simulink model "saturn_ib_stack_test"  (Simulink 6.2)
settings: Solver=ode4  SolverMode=SingleTasking  StartTime=-20.0  StopTime=620  FixedStep=0.005  RelTol=1e-3
values from neighbouring files (symbols this model uses):
  A_z_deg = 82.8200    (= 82.82)    [AS205_presettings.m]
  BN_1_sec = 14.4    [AS205_presettings.m]
  DeltaV_b_mps = 7.2381    [AS205_presettings.m]
  epsilon_2_sec = 15.0    (= 15)    [AS205_presettings.m]
  epsilon_prime_sec = 3.0    (= 3)    [AS205_presettings.m]
  i_deg = 28.89597    [AS205_presettings.m]
  lambda_0_deg = 102.32900    (= 102.329)    [AS205_presettings.m]
  lambda_L_deg = -80.561141    [AS205_presettings.m]
  pad_roll_L_deg = 100.0    (= 100)    [AS205_presettings.m]
  phi_L_deg = 28.521963    [AS205_presettings.m]
  phi_L_prime_deg = 28.360795    [AS205_presettings.m]
  R_L_m = 6373385.0    (= 6373385)    [AS205_presettings.m]
  R_T_m = 6570774.0    (= 6570774)    [AS205_presettings.m]
  T3_FM_sec = 6.08    [AS205_presettings.m]
  T_HSL_sec = 5.0    (= 5)    [AS205_presettings.m]
  Theta_T_deg = 0.000    (= 0)    [AS205_presettings.m]
  V_T_mps = 7780.976    [AS205_presettings.m]
  Xdotdot_VGT_mps2 = -9.251    [AS205_presettings.m]
undefined symbols (not defined in the file or in its folder): e0_0, e1_0, e2_0, e3_0, m, s
libraries: simulink x99, aerolibconvert x83, aerolibutil x63, aerolibtransform2 x34, aerolibasang x2, aerolibatmos2 x2, aerolib6dofsys x2
(part 7 of 7)

== system saturn_ib_stack_test/Saturn_IB_Stack/Saturn Instrument Unit (IU)/LVDA / LVDC/LVDC Iterative Guidance Mode/Position Correction Terms ==
  note: Enable Chi-tilde steering mode when T_3_i countdown
      | is near cutoff.  This is described in EDD section
      | 4.4.2.4, "Terminal Steering and Cutoff".
  J_prime_3 : Inport  Port=1  LatchInput=off
  tau_3_sec : Inport  Port=2  LatchInput=off
  T_3_i_sec : Inport  Port=3  LatchInput=off
  L_1 : Inport  Port=4  LatchInput=off
  J_1 : Inport  Port=5  LatchInput=off
  T_1_i_sec : Inport  Port=6  LatchInput=off
  S_1 : Inport  Port=7  LatchInput=off
  P_1 : Inport  Port=8  LatchInput=off
  Q_1 : Inport  Port=9  LatchInput=off
  U_1 : Inport  Port=10  LatchInput=off
  R_V_bar_m : Inport  Port=11  LatchInput=off
  V_V_bar_mps : Inport  Port=12  LatchInput=off
  G_star_V_bar_mps2 : Inport  Port=13  LatchInput=off
  T_star : Inport  Port=14  LatchInput=off
  L_3 : Inport  Port=15  LatchInput=off
  DeltaL_3 : Inport  Port=16  LatchInput=off
  Chi_z_tilde : Inport  Port=17  LatchInput=off
  Chi_y_tilde : Inport  Port=18  LatchInput=off
  Compare To Constant : simulink/Logic and Bit Operations/Compare To Constant  relop=<=  const=epsilon_2_sec  LogicOutDataTypeMode=boolean  ZeroCross=off
  Ground : Ground
  "Position Correction Terms - part 1 K_3, K_4 (Eqns. 4.4.51-67)" : Subsystem
  "Position Correction Terms - part 2 K_1, K_2 (Eqns. 4.4.68-80)" : Subsystem
  Switch{,1..3} (4 alike) : Switch  Criteria=u2 ~= 0
  K_1 : Outport
  K_2 : Outport  Port=2
  K_3 : Outport  Port=3
  K_4 : Outport  Port=4
  L_y : Outport  Port=5
  C_2 : Outport  Port=6
  C_4 : Outport  Port=7
  wires:
  DeltaL_3/1 -> "Position Correction Terms - part 1 K_3, K_4 (Eqns. 4.4.51-67)"/2(Delta_L_3)
  J_prime_3/1 -> "Position Correction Terms - part 1 K_3, K_4 (Eqns. 4.4.51-67)"/1(J_prime_3)
  tau_3_sec/1 -> "Position Correction Terms - part 2 K_1, K_2 (Eqns. 4.4.68-80)"/12(tau_3_sec), "Position Correction Terms - part 1 K_3, K_4 (Eqns. 4.4.51-67)"/3(tau_3_sec)
  L_1/1 -> "Position Correction Terms - part 1 K_3, K_4 (Eqns. 4.4.51-67)"/5(L_1)
  J_1/1 -> "Position Correction Terms - part 1 K_3, K_4 (Eqns. 4.4.51-67)"/6(J_1)
  S_1/1 -> "Position Correction Terms - part 1 K_3, K_4 (Eqns. 4.4.51-67)"/8(S_1)
  L_3/1 -> "Position Correction Terms - part 1 K_3, K_4 (Eqns. 4.4.51-67)"/9(L_3), "Position Correction Terms - part 2 K_1, K_2 (Eqns. 4.4.68-80)"/11(L_3)
  Q_1/1 -> "Position Correction Terms - part 1 K_3, K_4 (Eqns. 4.4.51-67)"/10(Q_1)
  R_V_bar_m/1 -> "Position Correction Terms - part 2 K_1, K_2 (Eqns. 4.4.68-80)"/16(R_V_bar_m), "Position Correction Terms - part 1 K_3, K_4 (Eqns. 4.4.51-67)"/11(R_V_bar_m)
  V_V_bar_mps/1 -> "Position Correction Terms - part 1 K_3, K_4 (Eqns. 4.4.51-67)"/12(V_V_bar_mps), "Position Correction Terms - part 2 K_1, K_2 (Eqns. 4.4.68-80)"/17(V_V_bar_mps)
  T_star/1 -> "Position Correction Terms - part 2 K_1, K_2 (Eqns. 4.4.68-80)"/19(T_star), "Position Correction Terms - part 1 K_3, K_4 (Eqns. 4.4.51-67)"/14(T_star)
  G_star_V_bar_mps2/1 -> "Position Correction Terms - part 2 K_1, K_2 (Eqns. 4.4.68-80)"/18(G_star_V_bar_mps2), "Position Correction Terms - part 1 K_3, K_4 (Eqns. 4.4.51-67)"/13(G_star_V_bar_mps2)
  T_3_i_sec/1 -> "Position Correction Terms - part 1 K_3, K_4 (Eqns. 4.4.51-67)"/4(T_3_i_sec), "Position Correction Terms - part 2 K_1, K_2 (Eqns. 4.4.68-80)"/13(T_3_i_sec), [T_3_i]
  T_1_i_sec/1 -> "Position Correction Terms - part 1 K_3, K_4 (Eqns. 4.4.51-67)"/7(T_1_i_sec), "Position Correction Terms - part 2 K_1, K_2 (Eqns. 4.4.68-80)"/14(T_1_i_sec)
  Chi_z_tilde/1 -> "Position Correction Terms - part 2 K_1, K_2 (Eqns. 4.4.68-80)"/20(Chi_z_tilde), "Position Correction Terms - part 1 K_3, K_4 (Eqns. 4.4.51-67)"/15(Chi_z)
  "Position Correction Terms - part 2 K_1, K_2 (Eqns. 4.4.68-80)"/1(K_1) -> Switch2/3
  "Position Correction Terms - part 1 K_3, K_4 (Eqns. 4.4.51-67)"/7(Q_y) -> "Position Correction Terms - part 2 K_1, K_2 (Eqns. 4.4.68-80)"/7(Q_y)
  "Position Correction Terms - part 2 K_1, K_2 (Eqns. 4.4.68-80)"/2(K_2) -> Switch3/3
  "Position Correction Terms - part 1 K_3, K_4 (Eqns. 4.4.51-67)"/8(K_3) -> "Position Correction Terms - part 2 K_1, K_2 (Eqns. 4.4.68-80)"/9(K_3), Switch/3
  "Position Correction Terms - part 1 K_3, K_4 (Eqns. 4.4.51-67)"/9(K_4) -> "Position Correction Terms - part 2 K_1, K_2 (Eqns. 4.4.68-80)"/10(K_4), Switch1/3
  "Position Correction Terms - part 1 K_3, K_4 (Eqns. 4.4.51-67)"/1(J_3) -> "Position Correction Terms - part 2 K_1, K_2 (Eqns. 4.4.68-80)"/1(J_3)  "J_3"
  "Position Correction Terms - part 1 K_3, K_4 (Eqns. 4.4.51-67)"/2(S_3) -> "Position Correction Terms - part 2 K_1, K_2 (Eqns. 4.4.68-80)"/2(S_3)  "S_3"
  "Position Correction Terms - part 1 K_3, K_4 (Eqns. 4.4.51-67)"/3(Q_3) -> "Position Correction Terms - part 2 K_1, K_2 (Eqns. 4.4.68-80)"/3(Q_3)
  "Position Correction Terms - part 1 K_3, K_4 (Eqns. 4.4.51-67)"/4(L_y) -> "Position Correction Terms - part 2 K_1, K_2 (Eqns. 4.4.68-80)"/4(L_y), L_y/1  "L_y"
  "Position Correction Terms - part 1 K_3, K_4 (Eqns. 4.4.51-67)"/5(J_y) -> "Position Correction Terms - part 2 K_1, K_2 (Eqns. 4.4.68-80)"/5(J_y)
  "Position Correction Terms - part 1 K_3, K_4 (Eqns. 4.4.51-67)"/6(S_y) -> "Position Correction Terms - part 2 K_1, K_2 (Eqns. 4.4.68-80)"/6(S_y)
  P_1/1 -> "Position Correction Terms - part 2 K_1, K_2 (Eqns. 4.4.68-80)"/15(P_1)
  Chi_y_tilde/1 -> "Position Correction Terms - part 2 K_1, K_2 (Eqns. 4.4.68-80)"/8(Chi_y_tilde)
  U_1/1 -> "Position Correction Terms - part 2 K_1, K_2 (Eqns. 4.4.68-80)"/21(U_1)
  "Position Correction Terms - part 2 K_1, K_2 (Eqns. 4.4.68-80)"/3(C_2) -> C_2/1
  "Position Correction Terms - part 2 K_1, K_2 (Eqns. 4.4.68-80)"/4(C_4) -> C_4/1
  Ground/1 -> Switch/1, Switch1/1, Switch2/1, Switch3/1
  Switch/1 -> K_3/1
  Switch1/1 -> K_4/1
  [T_3_i] -> Compare To Constant/1
  Compare To Constant/1 -> Switch/2, Switch1/2, Switch2/2, Switch3/2
  Switch2/1 -> K_1/1
  Switch3/1 -> K_2/1

== system saturn_ib_stack_test/Saturn_IB_Stack/Saturn Instrument Unit (IU)/LVDA / LVDC/LVDC Iterative Guidance Mode/SMCY ==
  Chi_y : Inport  Port=1  LatchInput=off
  Xdotdot_m : Inport  Port=2  LatchInput=off
  Zdotdot_m : Inport  Port=3  LatchInput=off
  Enable : EnablePort
  Add17 : Sum  Inputs=+-  OutScaling=2^-10
  Add19 : Sum  OutScaling=2^-10
  Add20 : Sum  Inputs=+-  OutScaling=2^-10
  Chi_y_last : Memory  InheritSampleTime=on
  Chi_y_last2 : Memory  InheritSampleTime=on
  Constant9 : Constant  Value=delta_T_sec/pi
  Divide6 : Product  Inputs=**/  OutScaling=2^-10
  Gain1 : Gain  Gain=0.5
  Product18 : Product  RndMeth=Zero
  Product19 : Product  RndMeth=Zero
  SMCG (Y-Axis) : Gain  Gain=0.03
  SMCY : Memory  Orientation=left  InheritSampleTime=on
  Sum2 : Sum  Inputs=|++  SampleTime=1.6
  Sum5 : Sum  Inputs=++|
  Trigonometric Function6 : Trigonometry  Operator=tan
  pirads to radians : Gain  Gain=pi
  SMCY_rad : Outport
  wires:
  SMCY/1 -> Sum2/2, Add20/2
  Sum2/1 -> SMCY/1, pirads to radians/1
  Chi_y_last/1 -> Sum5/2, Chi_y_last2/1
  Chi_y_last2/1 -> Sum5/1
  SMCG (Y-Axis)/1 -> Sum2/1
  Add20/1 -> Trigonometric Function6/1
  Divide6/1 -> SMCG (Y-Axis)/1
  Trigonometric Function6/1 -> Product19/1, Product18/1
  Xdotdot_m/1 -> Add17/1, Product18/2
  Zdotdot_m/1 -> Add19/1, Product19/2
  Product18/1 -> Add19/2
  Product19/1 -> Add17/2
  Constant9/1 -> Divide6/1
  Add19/1 -> Divide6/2
  Add17/1 -> Divide6/3
  Sum5/1 -> Gain1/1
  Gain1/1 -> Add20/1
  Chi_y/1 -> Chi_y_last/1
  pirads to radians/1 -> SMCY_rad/1

== system saturn_ib_stack_test/Saturn_IB_Stack/Saturn Instrument Unit (IU)/LVDA / LVDC/LVDC Iterative Guidance Mode/SMCZ ==
  Chi_z : Inport  Port=1  LatchInput=off
  Ydotdot_m : Inport  Port=2  LatchInput=off
  FoverM : Inport  Port=3  LatchInput=off
  Enable : EnablePort
  Add16 : Sum  Inputs=+-  OutScaling=2^-10
  Add18 : Sum  Inputs=+-  OutScaling=2^-10
  Chi_z_last : Memory  InheritSampleTime=on
  Chi_z_last2 : Memory  InheritSampleTime=on
  Constant8 : Constant  Value=delta_T_sec/pi
  Divide5 : Product  Inputs=**/  OutScaling=2^-10
  Divide7 : Product  Inputs=**  OutScaling=2^-10
  Gain : Gain  Gain=0.5
  Math Function8 : Math  Operator=reciprocal  SaturateOnIntegerOverflow=on
  SMCG : Gain  Gain=0.03
  SMCZ : Memory  Orientation=left  InheritSampleTime=on
  SinCos2 : aerolibutil/SinCos
  Sum3 : Sum  Inputs=|++  SampleTime=1.6
  Sum4 : Sum  Inputs=++|
  pirads to radians : Gain  Gain=pi
  SMCZ_rad : Outport
  wires:
  SMCZ/1 -> Sum3/2, Add16/2
  Sum3/1 -> SMCZ/1, pirads to radians/1
  Chi_z_last2/1 -> Sum4/1
  Sum4/1 -> Gain/1
  SMCG/1 -> Sum3/1
  Gain/1 -> Add16/1
  Add16/1 -> SinCos2/1
  Chi_z_last/1 -> Chi_z_last2/1, Sum4/2
  Divide5/1 -> SMCG/1
  Constant8/1 -> Divide5/1
  SinCos2/2 -> Divide5/3
  Add18/1 -> Divide5/2
  SinCos2/1 -> Add18/1
  Divide7/1 -> Add18/2
  Math Function8/1 -> Divide7/2
  Chi_z/1 -> Chi_z_last/1
  Ydotdot_m/1 -> Divide7/1
  FoverM/1 -> Math Function8/1
  pirads to radians/1 -> SMCZ_rad/1

== system saturn_ib_stack_test/Saturn_IB_Stack/Saturn Instrument Unit (IU)/LVDA / LVDC/LVDC Iterative Guidance Mode/Vector Display2 ==
  In1 : Inport  Port=1  LatchInput=off
  Demux5 : Demux  Outputs=3
  R_V_X : Display
  R_V_Y : Display
  R_V_Z : Display
  wires:
  Demux5/1 -> R_V_X/1
  Demux5/2 -> R_V_Y/1
  Demux5/3 -> R_V_Z/1
  In1/1 -> Demux5/1

== system saturn_ib_stack_test/Saturn_IB_Stack/Saturn Instrument Unit (IU)/LVDA / LVDC/LVDC S-Frame Position & Velocity Calculations/Estimated Gravitational Acceleration (Eqns. 4.3.6-12) ==
  note: Eqn. 4.3.6
  note: Eqn. 4.3.7
  note: Eqn. 4.3.12
  note: Eqn. 4.3.10
  note: Eqn. 4.3.11
  note: Mux outputs:
      | u(1)  X_S
      | u(2)  Y_S
      | u(3)  Z_S
      | u(4)  Y_G_bar
      | u(5)  R_m
      | u(6)  a_e/R_m
      | u(7)  Y_G/R_m
  XYZ_S_m : Inport  Port=1  LatchInput=off
  A_z_deg : Inport  Port=2  LatchInput=off
  phi_L_deg : Inport  Port=3  LatchInput=off
  2J : Gain  Gain=2.0*J
  Add : Sum  OutScaling=2^-10
  Add1 : Sum  OutScaling=2^-10
  Add2 : Sum  OutScaling=2^-10
  Angle Conversion : aerolibconvert/Angle Conversion  IU=deg  OU=rad
  Angle Conversion1 : aerolibconvert/Angle Conversion  IU=deg  OU=rad
  Constant : Constant  Value=-mu  OutDataTypeMode=double
  Constant1 : Constant  Value=-mu  OutDataTypeMode=double
  Divide : Product  Inputs=*/  OutScaling=2^-10
  Divide1 : Product  Inputs=*/  OutScaling=2^-10
  Divide2 : Product  Inputs=***/  OutScaling=2^-10
  Math Function : Math  Operator=square  SaturateOnIntegerOverflow=on
  Mux : Mux  Inputs=5
  Mux1 : Mux  Inputs=5
  Mux2 : Mux  Inputs=3
  P_34 : Fcn  Expr=H*u(6)*(15.0*u(7)^2-3.0) + (D/7.0)*u(6)^2*u(7)*(12.0-28.0*u(7)^2)
  Product : Product  RndMeth=Zero
  Product1 : Product  RndMeth=Zero
  Product2 : Product  RndMeth=Zero
  R^2 : Fcn  Expr=u(1)^2
  R^3 : Fcn  Expr=u(1)^3
  R_m : Fcn  Expr=sqrt(u(1)^2+u(2)^2+u(3)^2)
  S_34 : Fcn  Expr=H*u(6)^3*u(7)*(3-7*u(7)^2)+(D/7.0)*u(6)^4*(3.0-42*u(7)^2+63*u(7)^4)
  S_term : Fcn  Expr=1.0 + J*u(6)^2*(1.0-5.0*u(7)^2)
  SinCos1 : aerolibutil/SinCos
  SinCos2 : aerolibutil/SinCos
  X : Fcn  Expr=-u(6)
  Y : Fcn  Expr=u(7)*u(4)
  Y1 : Fcn  Expr=-u(7)*u(5)
  Y_G : Fcn  Expr=-u(1)*u(6)+u(2)*u(7)*u(4)-u(3)*u(7)*u(5)
  aaa : Fcn  Expr=a_e_m/u(1)
  Y_G_m : Outport
  G_S_bar_mps2 : Outport  Port=2  PortDimensions=3
  wires:
  A_z_deg/1 -> Angle Conversion/1
  Angle Conversion/1 -> SinCos1/1
  phi_L_deg/1 -> Angle Conversion1/1
  Angle Conversion1/1 -> SinCos2/1
  XYZ_S_m/1 -> Mux/1, Mux1/1, Product2/1
  SinCos1/1 -> Mux/2
  SinCos1/2 -> Mux/3
  SinCos2/1 -> Mux/4
  SinCos2/2 -> Mux/5
  Mux/1 -> Y_G/1, R_m/1, X/1, Y/1, Y1/1
  Y_G/1 -> Y_G_m/1, Mux1/2, Divide/1
  R_m/1 -> Mux1/3, Divide/2, R^3/1, R^2/1, aaa/1
  Mux1/1 -> P_34/1, S_term/1, S_34/1
  aaa/1 -> Mux1/4, Math Function/1
  Divide/1 -> Mux1/5, 2J/1
  Constant/1 -> Divide1/1
  R^3/1 -> Divide1/2
  S_term/1 -> Add/2
  Add/1 -> Product/1
  Divide1/1 -> Product/2
  Constant1/1 -> Divide2/1
  Math Function/1 -> Divide2/2
  X/1 -> Mux2/1
  Y/1 -> Mux2/2
  Y1/1 -> Mux2/3
  Mux2/1 -> Product1/2
  Divide2/1 -> Product1/1  "P"
  Product/1 -> Product2/2  "S"
  Product2/1 -> Add1/1
  Product1/1 -> Add1/2
  Add1/1 -> G_S_bar_mps2/1
  R^2/1 -> Divide2/4
  Add2/1 -> Divide2/3
  2J/1 -> Add2/1
  P_34/1 -> Add2/2
  S_34/1 -> Add/1

== system saturn_ib_stack_test/Saturn_IB_Stack/Saturn Instrument Unit (IU)/LVDA / LVDC/LVDC S-Frame Position & Velocity Calculations/Initial Position and Velocity (Eqns. 3.4.3-4) ==
  R_L_m : Inport  Port=1  PortDimensions=1  LatchInput=off
  A_z_deg : Inport  Port=2  LatchInput=off
  phi_L_deg : Inport  Port=3  LatchInput=off
  phi_L_prime_deg : Inport  Port=4  LatchInput=off
  Add : Sum  Inputs=+-  OutScaling=2^-10
  Angle Conversion : aerolibconvert/Angle Conversion  IU=deg  OU=rad
  Angle Conversion1 : aerolibconvert/Angle Conversion  IU=deg  OU=rad
  Angle Conversion2 : aerolibconvert/Angle Conversion  IU=deg  OU=rad
  Fcn : Fcn  Expr=u(1)*u(7)
  Fcn1 : Fcn  Expr=u(1)*u(6)*u(2)
  Fcn2 : Fcn  Expr=-u(1)*u(6)*u(3)
  Fcn3 : Fcn  Expr=0.0
  Fcn4 : Fcn  Expr=u(1)*omega_E_rps*pi*u(9)*u(3)
  Fcn5 : Fcn  Expr=u(1)*omega_E_rps*pi*u(9)*u(2)
  Mux : Mux  Inputs=9
  Mux1 : Mux  Inputs=3
  Mux2 : Mux  Inputs=3
  SinCos{1..4} (4 alike) : aerolibutil/SinCos
  R_S_0_m : Outport
  V_S_0_mps : Outport  Port=2
  wires:
  A_z_deg/1 -> Angle Conversion/1
  Angle Conversion/1 -> SinCos1/1
  phi_L_deg/1 -> Angle Conversion1/1
  Angle Conversion1/1 -> SinCos2/1, Add/1
  R_L_m/1 -> Mux/1
  SinCos1/1 -> Mux/2
  SinCos1/2 -> Mux/3
  SinCos2/1 -> Mux/4
  SinCos2/2 -> Mux/5
  phi_L_prime_deg/1 -> Angle Conversion2/1
  Angle Conversion2/1 -> Add/2, SinCos4/1
  Add/1 -> SinCos3/1
  SinCos3/1 -> Mux/6
  SinCos3/2 -> Mux/7
  Fcn/1 -> Mux1/1
  Fcn1/1 -> Mux1/2
  Fcn2/1 -> Mux1/3
  Mux/1 -> Fcn/1, Fcn1/1, Fcn2/1, Fcn3/1, Fcn4/1, Fcn5/1
  Mux1/1 -> R_S_0_m/1
  Fcn3/1 -> Mux2/1
  Fcn4/1 -> Mux2/2
  Fcn5/1 -> Mux2/3
  Mux2/1 -> V_S_0_mps/1
  SinCos4/1 -> Mux/8
  SinCos4/2 -> Mux/9

== system saturn_ib_stack_test/Saturn_IB_Stack/Saturn Instrument Unit (IU)/LVDA / LVDC/LVDC S-Frame Position & Velocity Calculations/Position and Velocity Calculation (S-Frame) (Eqns. 4.3.1-5) ==
  note: Eqn. 4.2.10
  note: Eqn 4.2.9
  note: This needs to be revised to
      | compute outputs more closely
      | based on the EDD.
  XYZdot_m_mps : Inport  Port=1  SampleTime=1.6  LatchInput=off
  XYZdotdot_Sg_mps2 : Inport  Port=2  LatchInput=off
  XYZ_0_m : Inport  Port=3  LatchInput=off
  XYZdot_0_mps : Inport  Port=4  LatchInput=off
  Delta_T_sec : Inport  Port=5  LatchInput=off
  TGRR_bias_sec : Inport  Port=6  LatchInput=off
  Gain3 : Gain  Gain=1 / delta_T_sec
  Math Function3 : Math  Operator=sqrt  SaturateOnIntegerOverflow=on
  Math Function4 : Math  Operator=square  SaturateOnIntegerOverflow=on
  Memory2 : Memory  X0=[-0.5 0.0 0.0]  InheritSampleTime=on
  Product18 : Product  Multiplication=Matrix(*)  RndMeth=Zero
  Product6 : Product  Multiplication=Matrix(*)  RndMeth=Zero
  Sum : Sum  Inputs=|+-
  Sum of Elements1 : Sum  Inputs=+  OutScaling=2^-10
  Switch{1..3,5} (4 alike) : Switch  Criteria=u2 ~= 0
  T_1_i_sec : DataStoreMemory  DataStoreName=XYZdot_Sg_mps  InitialValue=[0.0 0.0 0.0]  DataType=double
  Terminator{,1..4} (5 alike) : Terminator
  tau_1_sec : DataStoreMemory  DataStoreName=XYZ_S_m  InitialValue=[0.0 0.0 0.0]  DataType=double
  XYZ_S_m : Outport  SampleTime=1.6
  XYZdot_S_mps : Outport  Port=2  PortDimensions=3  SampleTime=1.6
  A_m_bar_mps2 : Outport  Port=3  PortDimensions=3  SampleTime=1.6
  FoverM_mps2 : Outport  Port=4  PortDimensions=1  SampleTime=1.6
  wires:
  XYZdotdot_Sg_mps2/1 -> Terminator4/1
  XYZdot_m_mps/1 -> Memory2/1, Sum/1
  Sum of Elements1/1 -> Math Function3/1
  Math Function4/1 -> Sum of Elements1/1
  Math Function3/1 -> FoverM_mps2/1
  Memory2/1 -> Sum/2
  Sum/1 -> Gain3/1
  Gain3/1 -> Math Function4/1, A_m_bar_mps2/1
  [S_IVB_Xe_m] -> Switch5/1
  [bStageSep] -> Switch5/2
  Switch5/1 -> Product18/2
  [MES_DCM] -> Product18/1
  Product18/1 -> XYZ_S_m/1
  [S_IVB_Ve_mps] -> Switch1/1
  [bStageSep] -> Switch1/2
  Switch1/1 -> Product6/2
  [MES_DCM] -> Product6/1
  Product6/1 -> XYZdot_S_mps/1
  XYZ_0_m/1 -> Terminator/1
  TGRR_bias_sec/1 -> Terminator1/1
  XYZdot_0_mps/1 -> Terminator2/1
  Delta_T_sec/1 -> Terminator3/1
  Switch3/1 -> Switch5/3
  [bLiftoff] -> Switch3/2
  [bLiftoff] -> Switch2/2
  Switch2/1 -> Switch1/3
  [Xe_m] -> Switch3/1
  [PAD_Xe_m] -> Switch3/3
  [PAD_Ve_mps] -> Switch2/3
  [Ve_mps] -> Switch2/1

== system saturn_ib_stack_test/Saturn_IB_Stack/Saturn Instrument Unit (IU)/LVDA / LVDC/LVDC S-Frame Position & Velocity Calculations/Reciprocal Acceleration Filter (EDD eqn. 4.2.11) ==
  A_S_mps2 : Inport  Port=1  DataType=double  LatchInput=off
  Enable : EnablePort
  +/- 0.25 sec^2/m : Saturate  UpperLimit=inf  LowerLimit=4.00
  MF2 : Memory  X0=0.135  InheritSampleTime=on
  MF3 : Memory  X0=0.135  InheritSampleTime=on
  MF4 : Memory  X0=0.135  InheritSampleTime=on
  MFK : Constant  Value=[0.0120948 0.0213339 -0.0261577 -0.00526684 2.80483 -2.85880 1.24933 -0.197360]
  MFS{1..4} (4 alike) : Memory  X0=0.135  InheritSampleTime=on
  Math Function5 : Math  Operator=reciprocal  SaturateOnIntegerOverflow=on
  Mux1 : Mux  Inputs=8
  Product1 : Product  RndMeth=Zero
  Sum of Elements : Sum  Inputs=+  OutScaling=2^-10
  MF_S : Outport
  wires:
  MFS2/1 -> MFS3/1, Mux1/6
  MFS1/1 -> MFS2/1, Mux1/5
  MFS3/1 -> MFS4/1, Mux1/7
  MF2/1 -> MF3/1, Mux1/2
  MF3/1 -> MF4/1, Mux1/3
  Mux1/1 -> Product1/1
  MFK/1 -> Product1/2
  Product1/1 -> Sum of Elements/1
  MF4/1 -> Mux1/4
  MFS4/1 -> Mux1/8
  Sum of Elements/1 -> MFS1/1, MF_S/1
  A_S_mps2/1 -> +/- 0.25 sec^2/m/1
  Math Function5/1 -> MF2/1, Mux1/1
  +/- 0.25 sec^2/m/1 -> Math Function5/1

== system saturn_ib_stack_test/Saturn_IB_Stack/Saturn Instrument Unit (IU)/LVDA / LVDC/T1 Timer/Timer Initialization ==
  In1 : Inport  Port=1  LatchInput=off
  Trigger : TriggerPort
  Data Store Write : DataStoreWrite  DataStoreName=A  SampleTime=-1
  wires:
  In1/1 -> Data Store Write/1

== system saturn_ib_stack_test/Saturn_IB_Stack/Saturn Instrument Unit (IU)/LVDA / LVDC/T2 Timer/Timer Initialization ==
  In1 : Inport  Port=1  LatchInput=off
  Trigger : TriggerPort
  Data Store Write : DataStoreWrite  DataStoreName=A  SampleTime=-1
  wires:
  In1/1 -> Data Store Write/1

== system saturn_ib_stack_test/Saturn_IB_Stack/Saturn Instrument Unit (IU)/LVDA / LVDC/T3 Timer/Timer Initialization ==
  In1 : Inport  Port=1  LatchInput=off
  Trigger : TriggerPort
  Data Store Write : DataStoreWrite  DataStoreName=A  SampleTime=-1
  wires:
  In1/1 -> Data Store Write/1

== system saturn_ib_stack_test/Saturn_IB_Stack/Saturn Instrument Unit (IU)/LVDA / LVDC/T4 Timer/Timer Initialization ==
  In1 : Inport  Port=1  LatchInput=off
  Trigger : TriggerPort
  Data Store Write : DataStoreWrite  DataStoreName=A  SampleTime=-1
  wires:
  In1/1 -> Data Store Write/1

== system saturn_ib_stack_test/Saturn_IB_Stack/On Pad/Initial Conditions/MES Transform/MES Transform/E-Frame to s-Frame (MES matrix) ==
  note: u(1)  sin Az
      | u(2)  sin Phi_L
      | u(3)  sin Theta_E
      | u(4)  cos Az
      | u(5)  cos Phi_L
      | u(6)  cos Theta_E
  note: Eqn 2.3.10
  Az phi_L Theta_E : Inport  Port=1  LatchInput=off
  11 : Fcn  Expr=u(5)*u(6)
  12 : Fcn  Expr=u(5)*u(3)
  13 : Fcn  Expr=u(2)
  21 : Fcn  Expr=u(2)*u(1)*u(6)-u(4)*u(3)
  22 : Fcn  Expr=u(2)*u(1)*u(3)+u(4)*u(6)
  23 : Fcn  Expr=-u(5)*u(1)
  31 : Fcn  Expr=-u(2)*u(4)*u(6)-u(1)*u(3)
  32 : Fcn  Expr=-u(2)*u(4)*u(3)+u(1)*u(6)
  33 : Fcn  Expr=u(5)*u(4)
  Mux : Mux  Inputs=2
  Mux2 : Mux  Inputs=9
  Reshape 9x1->3x3 : simulink/Math Operations/Reshape  OutputDimensionality=Customize  OutputDimensions=[3,3]
  SinCos3 : aerolibutil/SinCos
  DCM : Outport  InitialOutput=0
  wires:
  33/1 -> Mux2/9
  22/1 -> Mux2/5
  11/1 -> Mux2/1
  Mux2/1 -> Reshape 9x1->3x3/1
  Reshape 9x1->3x3/1 -> DCM/1
  Mux/1 -> 22/1, 11/1, 21/1, 31/1, 12/1, 32/1, 13/1, 33/1, 23/1
  23/1 -> Mux2/8
  13/1 -> Mux2/7
  32/1 -> Mux2/6
  12/1 -> Mux2/4
  31/1 -> Mux2/3
  21/1 -> Mux2/2
  Az phi_L Theta_E/1 -> SinCos3/1
  SinCos3/1 -> Mux/1
  SinCos3/2 -> Mux/2

== system saturn_ib_stack_test/Saturn_IB_Stack/S-IB Stage/H-1 Engine Cluster/Engine 1/Triggered Timer/Timer Initialization ==
  In1 : Inport  Port=1  LatchInput=off
  Trigger : TriggerPort
  Data Store Write : DataStoreWrite  DataStoreName=A  SampleTime=-1
  wires:
  In1/1 -> Data Store Write/1

== system saturn_ib_stack_test/Saturn_IB_Stack/S-IB Stage/H-1 Engine Cluster/Engine 2/Triggered Timer/Timer Initialization ==
  In1 : Inport  Port=1  LatchInput=off
  Trigger : TriggerPort
  Data Store Write : DataStoreWrite  DataStoreName=A  SampleTime=-1
  wires:
  In1/1 -> Data Store Write/1

== system saturn_ib_stack_test/Saturn_IB_Stack/S-IB Stage/H-1 Engine Cluster/Engine 3/Triggered Timer/Timer Initialization ==
  In1 : Inport  Port=1  LatchInput=off
  Trigger : TriggerPort
  Data Store Write : DataStoreWrite  DataStoreName=A  SampleTime=-1
  wires:
  In1/1 -> Data Store Write/1

== system saturn_ib_stack_test/Saturn_IB_Stack/S-IB Stage/H-1 Engine Cluster/Engine 4/Triggered Timer/Timer Initialization ==
  In1 : Inport  Port=1  LatchInput=off
  Trigger : TriggerPort
  Data Store Write : DataStoreWrite  DataStoreName=A  SampleTime=-1
  wires:
  In1/1 -> Data Store Write/1

== system saturn_ib_stack_test/Saturn_IB_Stack/S-IB Stage/H-1 Engine Cluster/Engine 5/Triggered Timer/Timer Initialization ==
  In1 : Inport  Port=1  LatchInput=off
  Trigger : TriggerPort
  Data Store Write : DataStoreWrite  DataStoreName=A  SampleTime=-1
  wires:
  In1/1 -> Data Store Write/1

== system saturn_ib_stack_test/Saturn_IB_Stack/S-IB Stage/H-1 Engine Cluster/Engine 6/Triggered Timer/Timer Initialization ==
  In1 : Inport  Port=1  LatchInput=off
  Trigger : TriggerPort
  Data Store Write : DataStoreWrite  DataStoreName=A  SampleTime=-1
  wires:
  In1/1 -> Data Store Write/1

== system saturn_ib_stack_test/Saturn_IB_Stack/S-IB Stage/H-1 Engine Cluster/Engine 7/Triggered Timer/Timer Initialization ==
  In1 : Inport  Port=1  LatchInput=off
  Trigger : TriggerPort
  Data Store Write : DataStoreWrite  DataStoreName=A  SampleTime=-1
  wires:
  In1/1 -> Data Store Write/1

== system saturn_ib_stack_test/Saturn_IB_Stack/S-IB Stage/H-1 Engine Cluster/Engine 8/Triggered Timer/Timer Initialization ==
  In1 : Inport  Port=1  LatchInput=off
  Trigger : TriggerPort
  Data Store Write : DataStoreWrite  DataStoreName=A  SampleTime=-1
  wires:
  In1/1 -> Data Store Write/1

== system saturn_ib_stack_test/Saturn_IB_Stack/S-IVB Stage/J-2 Engine/Thrust Model/Time Since Engine Start/Timer Initialization ==
  In1 : Inport  Port=1  LatchInput=off
  Trigger : TriggerPort
  Data Store Write : DataStoreWrite  DataStoreName=A  SampleTime=-1
  wires:
  In1/1 -> Data Store Write/1

== system saturn_ib_stack_test/Saturn_IB_Stack/S-IVB Stage/J-2 Engine/Thrust Model/Time Since Shutdown/Timer Initialization ==
  In1 : Inport  Port=1  LatchInput=off
  Trigger : TriggerPort
  Data Store Write : DataStoreWrite  DataStoreName=A  SampleTime=-1
  wires:
  In1/1 -> Data Store Write/1

== system saturn_ib_stack_test/Saturn_IB_Stack/Saturn Instrument Unit (IU)/LVDA / LVDC/LVDC Iterative Guidance Mode/IGM First Phase/Set nIGMMode to "1" ==
  note: Switch mode for next BML to first cycle in Phase 2
      | (nIGMMode = 1)
  Action Port : ActionPort  ActionType=then
  Data Store Write : DataStoreWrite  DataStoreName=nIGMMode  SampleTime=-1
  First BML of Phase 2 : Constant  OutDataTypeMode=int8
  wires:
  First BML of Phase 2/1 -> Data Store Write/1

== system saturn_ib_stack_test/Saturn_IB_Stack/Saturn Instrument Unit (IU)/LVDA / LVDC/LVDC Iterative Guidance Mode/IGM Phase2 (HSL first pass)/Set HSL Mode ==
  Action Port : ActionPort  ActionType=then
  Data Store Write : DataStoreWrite  DataStoreName=nHSLActive  SampleTime=-1
  "HSL mode \"ON\"" : Constant  OutDataTypeMode=int32
  wires:
  "HSL mode \"ON\""/1 -> Data Store Write/1

== system saturn_ib_stack_test/Saturn_IB_Stack/Saturn Instrument Unit (IU)/LVDA / LVDC/LVDC Iterative Guidance Mode/IGM Phase2 (artificial tau complete)/Set HSL Mode ==
  Action Port : ActionPort  ActionType=then
  Data Store Write : DataStoreWrite  DataStoreName=nIGMMode  SampleTime=-1
  "HSL mode \"ON\"" : Constant  Value=4  OutDataTypeMode=int8
  wires:
  "HSL mode \"ON\""/1 -> Data Store Write/1

== system saturn_ib_stack_test/Saturn_IB_Stack/Saturn Instrument Unit (IU)/LVDA / LVDC/LVDC Iterative Guidance Mode/IGM Phase2 (artificial tau complete)/Set Terminal Steering Mode ==
  Action Port : ActionPort  ActionType=then
  Data Store Write : DataStoreWrite  DataStoreName=nTerminalSteeringMode  SampleTime=-1
  "terminal steering mode \"ON\"" : Constant  OutDataTypeMode=int8
  wires:
  "terminal steering mode \"ON\""/1 -> Data Store Write/1

== system saturn_ib_stack_test/Saturn_IB_Stack/Saturn Instrument Unit (IU)/LVDA / LVDC/LVDC Iterative Guidance Mode/IGM Phase2 (artificial tau mode)/Set nIGMMode to "3" ==
  Action Port : ActionPort  ActionType=then
  Data Store Write : DataStoreWrite  DataStoreName=nIGMMode  SampleTime=-1
  artifical tau complete : Constant  Value=3  OutDataTypeMode=int8
  wires:
  artifical tau complete/1 -> Data Store Write/1

== system saturn_ib_stack_test/Saturn_IB_Stack/Saturn Instrument Unit (IU)/LVDA / LVDC/LVDC Iterative Guidance Mode/MS4 Transform Matrix/S-Frame to 4-Frame (MS4 matrix) ==
  note: u(1)  sin Az
      | u(2)  sin phi_L
      | u(3)  sin lambda
      | u(4)  cos Az
      | u(5)  cos phi_L
      | u(6)  cos lambda
      | u(7)  sin i
      | u(8)  cos i
  Az phi_L lambda : Inport  Port=1  LatchInput=off
  i_rad : Inport  Port=2  LatchInput=off
  11 : Fcn  Expr=u(6)*u(5)
  12 : Fcn  Expr=u(6)*u(2)*u(1)+u(3)*u(4)
  13 : Fcn  Expr=-u(6)*u(2)*u(4)+u(3)*u(1)
  21 : Fcn  Expr=u(7)*u(3)*u(5)-u(8)*u(2)
  22 : Fcn  Expr=u(7)*u(3)*u(2)*u(1)+u(8)*u(5)*u(1)-u(7)*u(6)*u(4)
  23 : Fcn  Expr=-u(7)*u(3)*u(2)*u(4)-u(8)*u(5)*u(4)-u(7)*u(6)*u(1)
  31 : Fcn  Expr=-u(8)*u(3)*u(5)-u(7)*u(2)
  32 : Fcn  Expr=-u(8)*u(3)*u(2)*u(1)+u(7)*u(5)*u(1)+u(8)*u(6)*u(4)
  33 : Fcn  Expr=u(8)*u(3)*u(2)*u(4)-u(7)*u(5)*u(4)+u(8)*u(6)*u(1)
  Demux : Demux  Outputs=3
  Mux : Mux  Inputs=8
  Mux2 : Mux  Inputs=9
  Reshape 9x1->3x3 : simulink/Math Operations/Reshape  OutputDimensionality=Customize  OutputDimensions=[3,3]
  SinCos{,1..3} (4 alike) : aerolibutil/SinCos
  DCM : Outport  InitialOutput=0
  wires:
  33/1 -> Mux2/9
  22/1 -> Mux2/5
  11/1 -> Mux2/1
  Mux2/1 -> Reshape 9x1->3x3/1
  Reshape 9x1->3x3/1 -> DCM/1
  Mux/1 -> 22/1, 11/1, 21/1, 31/1, 12/1, 32/1, 13/1, 33/1, 23/1
  i_rad/1 -> SinCos1/1
  23/1 -> Mux2/8
  13/1 -> Mux2/7
  32/1 -> Mux2/6
  12/1 -> Mux2/4
  31/1 -> Mux2/3
  21/1 -> Mux2/2
  Az phi_L lambda/1 -> Demux/1
  SinCos3/1 -> Mux/1
  Demux/1 -> SinCos3/1
  Demux/2 -> SinCos2/1
  Demux/3 -> SinCos/1
  SinCos1/2 -> Mux/8
  SinCos1/1 -> Mux/7
  SinCos2/1 -> Mux/2
  SinCos/1 -> Mux/3
  SinCos/2 -> Mux/6
  SinCos2/2 -> Mux/5
  SinCos3/2 -> Mux/4

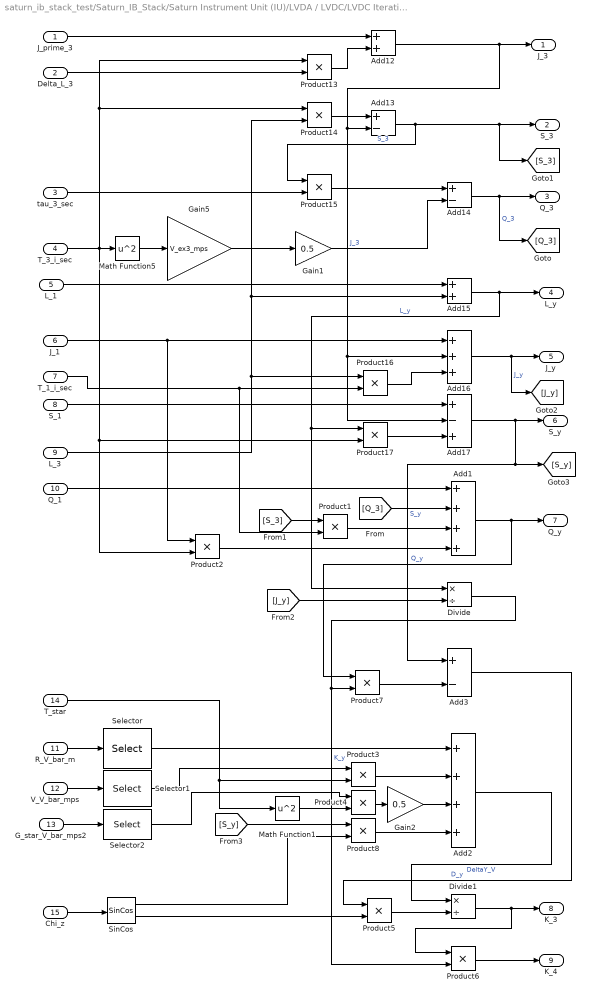
== system saturn_ib_stack_test/Saturn_IB_Stack/Saturn Instrument Unit (IU)/LVDA / LVDC/LVDC Iterative Guidance Mode/Position Correction Terms/Position Correction Terms - part 1 K_3, K_4 (Eqns. 4.4.51-67) ==
  J_prime_3 : Inport  Port=1  LatchInput=off
  Delta_L_3 : Inport  Port=2  LatchInput=off
  tau_3_sec : Inport  Port=3  LatchInput=off
  T_3_i_sec : Inport  Port=4  LatchInput=off
  L_1 : Inport  Port=5  LatchInput=off
  J_1 : Inport  Port=6  LatchInput=off
  T_1_i_sec : Inport  Port=7  LatchInput=off
  S_1 : Inport  Port=8  LatchInput=off
  L_3 : Inport  Port=9  LatchInput=off
  Q_1 : Inport  Port=10  LatchInput=off
  R_V_bar_m : Inport  Port=11  LatchInput=off
  V_V_bar_mps : Inport  Port=12  LatchInput=off
  G_star_V_bar_mps2 : Inport  Port=13  LatchInput=off
  T_star : Inport  Port=14  LatchInput=off
  Chi_z : Inport  Port=15  LatchInput=off
  Add1 : Sum  Inputs=++++  OutScaling=2^-10
  Add12 : Sum  OutScaling=2^-10
  Add13 : Sum  Inputs=+-  OutScaling=2^-10
  Add14 : Sum  Inputs=+-  OutScaling=2^-10
  Add15 : Sum  OutScaling=2^-10
  Add16 : Sum  Inputs=+++  OutScaling=2^-10
  Add17 : Sum  Inputs=+-+  OutScaling=2^-10
  Add2 : Sum  Inputs=++++  OutScaling=2^-10
  Add3 : Sum  Inputs=+-  OutScaling=2^-10
  Divide : Product  Inputs=*/  OutScaling=2^-10
  Divide1 : Product  Inputs=*/  OutScaling=2^-10
  Gain1 : Gain  Gain=0.5
  Gain2 : Gain  Gain=0.5
  Gain5 : Gain  Gain=V_ex3_mps
  Math Function1 : Math  Operator=square  SaturateOnIntegerOverflow=on
  Math Function5 : Math  Operator=square  SaturateOnIntegerOverflow=on
  Product{1..8,13..17} (13 alike) : Product  RndMeth=Zero
  Selector : Selector  Elements=[2]  InputPortWidth=3
  Selector1 : Selector  Elements=[2]  InputPortWidth=3
  Selector2 : Selector  Elements=[2]  InputPortWidth=3
  SinCos : aerolibutil/SinCos
  J_3 : Outport
  S_3 : Outport  Port=2
  Q_3 : Outport  Port=3
  L_y : Outport  Port=4
  J_y : Outport  Port=5
  S_y : Outport  Port=6
  Q_y : Outport  Port=7
  K_3 : Outport  Port=8
  K_4 : Outport  Port=9
  wires:
  Product13/1 -> Add12/2
  Add12/1 -> Add13/2, Add16/2, Add17/2, J_3/1  "J_3"
  L_3/1 -> Product16/1, Add15/2, Product14/2
  Product14/1 -> Add13/1
  Add13/1 -> Product15/1, S_3/1, [S_3]  "S_3"
  Product15/1 -> Add14/1
  Math Function5/1 -> Gain5/1
  Gain5/1 -> Gain1/1
  Gain1/1 -> Add14/2
  Add15/1 -> L_y/1, Product17/1, Divide/1  "L_y"
  Product16/1 -> Add16/3
  Product17/1 -> Add17/3
  T_3_i_sec/1 -> Product13/1, Product14/1, Math Function5/1, Product17/2, Product2/2
  T_1_i_sec/1 -> Product16/2, Product1/2
  J_prime_3/1 -> Add12/1
  Delta_L_3/1 -> Product13/2
  tau_3_sec/1 -> Product15/2
  Add14/1 -> Q_3/1, [Q_3]  "Q_3"
  L_1/1 -> Add15/1
  J_1/1 -> Add16/1, Product2/1
  Add16/1 -> J_y/1, [J_y]  "J_y"
  S_1/1 -> Add17/1
  Add17/1 -> S_y/1, Add3/1, [S_y]  "S_y"
  Q_1/1 -> Add1/1
  [Q_3] -> Add1/2
  Product1/1 -> Add1/3
  [S_3] -> Product1/1
  Product2/1 -> Add1/4
  Add1/1 -> Q_y/1, Product7/1  "Q_y"
  [J_y] -> Divide/2
  Divide/1 -> Product7/2, Product6/2  "K_y"
  R_V_bar_m/1 -> Selector/1
  V_V_bar_mps/1 -> Selector1/1
  G_star_V_bar_mps2/1 -> Selector2/1
  Selector/1 -> Add2/1
  Product3/1 -> Add2/2
  Selector1/1 -> Product3/1
  T_star/1 -> Product3/2, Math Function1/1
  Product4/1 -> Gain2/1
  Gain2/1 -> Add2/3
  Selector2/1 -> Product4/1
  Math Function1/1 -> Product4/2
  Add2/1 -> Divide1/1  "DeltaY_V"
  Chi_z/1 -> SinCos/1
  Divide1/1 -> K_3/1, Product6/1
  Product5/1 -> Divide1/2
  SinCos/2 -> Product5/2
  Product6/1 -> K_4/1
  Product7/1 -> Add3/2
  Add3/1 -> Product5/1  "D_y"
  Product8/1 -> Add2/4
  SinCos/1 -> Product8/2
  [S_y] -> Product8/1

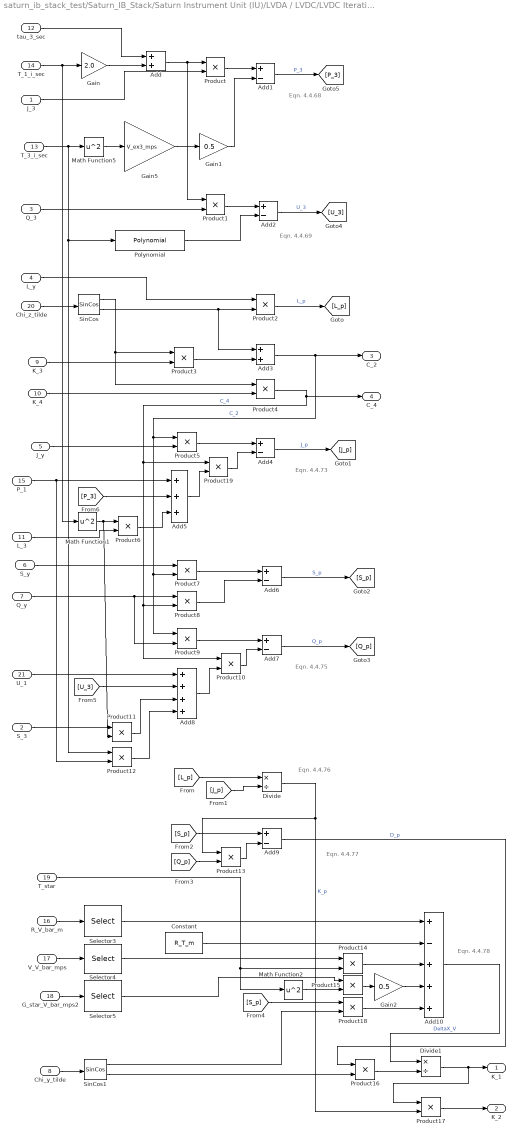
== system saturn_ib_stack_test/Saturn_IB_Stack/Saturn Instrument Unit (IU)/LVDA / LVDC/LVDC Iterative Guidance Mode/Position Correction Terms/Position Correction Terms - part 2 K_1, K_2 (Eqns. 4.4.68-80) ==
  note: Eqn. 4.4.78
  note: Eqn. 4.4.76
  note: Eqn. 4.4.77
  note: Eqn. 4.4.75
  note: Eqn. 4.4.73
  note: Eqn. 4.4.68
  note: Eqn. 4.4.69
  J_3 : Inport  Port=1  LatchInput=off
  S_3 : Inport  Port=2  LatchInput=off
  Q_3 : Inport  Port=3  LatchInput=off
  L_y : Inport  Port=4  LatchInput=off
  J_y : Inport  Port=5  LatchInput=off
  S_y : Inport  Port=6  LatchInput=off
  Q_y : Inport  Port=7  LatchInput=off
  Chi_y_tilde : Inport  Port=8  LatchInput=off
  K_3 : Inport  Port=9  LatchInput=off
  K_4 : Inport  Port=10  LatchInput=off
  L_3 : Inport  Port=11  LatchInput=off
  tau_3_sec : Inport  Port=12  LatchInput=off
  T_3_i_sec : Inport  Port=13  LatchInput=off
  T_1_i_sec : Inport  Port=14  LatchInput=off
  P_1 : Inport  Port=15  LatchInput=off
  R_V_bar_m : Inport  Port=16  LatchInput=off
  V_V_bar_mps : Inport  Port=17  LatchInput=off
  G_star_V_bar_mps2 : Inport  Port=18  LatchInput=off
  T_star : Inport  Port=19  LatchInput=off
  Chi_z_tilde : Inport  Port=20  LatchInput=off
  U_1 : Inport  Port=21  LatchInput=off
  Add : Sum  OutScaling=2^-10
  Add{1..2,4,6..7,9} (6 alike) : Sum  Inputs=+-  OutScaling=2^-10
  Add10 : Sum  Inputs=+-+++  OutScaling=2^-10
  Add3 : Sum  OutScaling=2^-10
  Add5 : Sum  Inputs=+++  OutScaling=2^-10
  Add8 : Sum  Inputs=++++  OutScaling=2^-10
  Constant : Constant  Value=R_T_m
  Divide : Product  Inputs=*/  OutScaling=2^-10
  Divide1 : Product  Inputs=*/  OutScaling=2^-10
  Gain : Gain  Gain=2.0
  Gain1 : Gain  Gain=0.5
  Gain2 : Gain  Gain=0.5
  Gain5 : Gain  Gain=V_ex3_mps
  Math Function1 : Math  Operator=square  SaturateOnIntegerOverflow=on
  Math Function2 : Math  Operator=square  SaturateOnIntegerOverflow=on
  Math Function5 : Math  Operator=square  SaturateOnIntegerOverflow=on
  Polynomial : simulink/Math Operations/Polynomial  coefs=[V_ex3_mps/6.0 0.0 0.0 0.0]
  Product{,1..19} (20 alike) : Product  RndMeth=Zero
  Selector3 : Selector  Elements=[1]  InputPortWidth=3
  Selector4 : Selector  Elements=[1]  InputPortWidth=3
  Selector5 : Selector  Elements=[1]  InputPortWidth=3
  SinCos : aerolibutil/SinCos
  SinCos1 : aerolibutil/SinCos
  K_1 : Outport
  K_2 : Outport  Port=2
  C_2 : Outport  Port=3
  C_4 : Outport  Port=4
  wires:
  R_V_bar_m/1 -> Selector3/1
  V_V_bar_mps/1 -> Selector4/1
  G_star_V_bar_mps2/1 -> Selector5/1
  Chi_z_tilde/1 -> SinCos/1
  T_1_i_sec/1 -> Gain/1, Math Function1/1
  Gain/1 -> Add/2
  tau_3_sec/1 -> Add/1
  Add/1 -> Product/1, Product1/1
  J_3/1 -> Product/2
  Product/1 -> Add1/1
  Math Function5/1 -> Gain5/1
  Gain5/1 -> Gain1/1
  T_3_i_sec/1 -> Math Function5/1, Polynomial/1, Product12/1
  Gain1/1 -> Add1/2
  Add1/1 -> [P_3]  "P_3"
  Q_3/1 -> Product1/2
  Product1/1 -> Add2/1
  Polynomial/1 -> Add2/2
  Add2/1 -> [U_3]  "U_3"
  L_y/1 -> Product2/1
  SinCos/2 -> Product2/2, Add3/1
  Product2/1 -> [L_p]  "L_p"
  SinCos/1 -> Product3/1, Product4/1
  K_3/1 -> Product3/2
  Product3/1 -> Add3/2
  Add3/1 -> Product5/1, Product7/2, Product9/1, C_2/1  "C_2"
  K_4/1 -> Product4/2
  Product4/1 -> Product8/2, Product10/1, Product19/1, C_4/1  "C_4"
  J_y/1 -> Product5/2
  Product5/1 -> Add4/1
  P_1/1 -> Add5/1, Product12/2
  Math Function1/1 -> Product6/1, Product11/2
  L_3/1 -> Product6/2
  Product6/1 -> Add5/3
  Add4/1 -> [J_p]  "J_p"
  S_y/1 -> Product7/1
  Product7/1 -> Add6/1
  Q_y/1 -> Product8/1, Product9/2
  Product8/1 -> Add6/2
  Add6/1 -> [S_p]  "S_p"
  Product9/1 -> Add7/1
  Product10/1 -> Add7/2
  U_1/1 -> Add8/1
  Add8/1 -> Product10/2
  Add7/1 -> [Q_p]  "Q_p"
  S_3/1 -> Product11/1
  Product11/1 -> Add8/3
  Product12/1 -> Add8/4
  [L_p] -> Divide/1
  [J_p] -> Divide/2
  Divide/1 -> Product13/1, Product17/2  "K_p"
  [S_p] -> Add9/1
  Product13/1 -> Add9/2
  Add9/1 -> Product16/1  "D_p"
  [Q_p] -> Product13/2
  Selector4/1 -> Product14/1
  T_star/1 -> Product14/2, Math Function2/1
  Product15/1 -> Gain2/1
  Selector5/1 -> Product15/1
  Math Function2/1 -> Product15/2
  Add10/1 -> Divide1/1  "DeltaX_V"
  Divide1/1 -> Product17/1, K_1/1
  Product16/1 -> Divide1/2
  Product17/1 -> K_2/1
  [S_p] -> Product18/1
  Chi_y_tilde/1 -> SinCos1/1
  SinCos1/1 -> Product18/2
  SinCos1/2 -> Product16/2
  [U_3] -> Add8/2
  [P_3] -> Add5/2
  Product18/1 -> Add10/5
  Gain2/1 -> Add10/4
  Product14/1 -> Add10/3
  Selector3/1 -> Add10/1
  Constant/1 -> Add10/2
  Product19/1 -> Add4/2
  Add5/1 -> Product19/2
